simulink model "DetailedModel"  (R2024b)
settings: Solver=ode23t  StartTime=0.0  StopTime=0.2  MaxStep=1e-6  RelTol=1e-4
InitFcn:
  | ModelParameters
undefined symbols (not defined in the file or in its folder): ABR, abr, dc, dc_vs, h_BTU, inv, L, setpoint, Setpoint_Harmonic_L1, time, ts, Ts_RMS
libraries: spsThreePhaseSeriesRLCBranchLib x17, spsGroundLib x14, spsControlledVoltageSourceLib x11, spsThreePhaseVIMeasurementLib x8, spsSeriesRLCBranchLib x7, eePwmGenerator x6, spsCurrentMeasurementLib x4, spsVoltageMeasurementLib x4, spsControlledCurrentSourceLib x3, eePowerMeasurement x3, spsUniversalBridgeLib x2, spsThreePhaseBreakerLib x1
(part 2 of 3)

== system DetailedModel/ powerline/ 10 km ==
  note: L1
  note: L2
  Ground : spsGroundLib/Ground  LConnTagsString=a
  Three-Phase Series RLC Branch1 : spsThreePhaseSeriesRLCBranchLib/Three-Phase Series RLC Branch  LConnTagsString=A|B|C  RConnTagsString=A|B|C  BranchType=RL  Resistance=R  Inductance=L  Capacitance=1e-6  Measurements=None
  Three-Phase Series RLC Branch2 : spsThreePhaseSeriesRLCBranchLib/Three-Phase Series RLC Branch  LConnTagsString=A|B|C  RConnTagsString=A|B|C  BranchType=C  Resistance=inv.RC  Inductance=13e-6  Capacitance=C  Measurements=None
  Three-Phase Series RLC Branch3 : spsThreePhaseSeriesRLCBranchLib/Three-Phase Series RLC Branch  LConnTagsString=A|B|C  RConnTagsString=A|B|C  BranchType=C  Resistance=inv.RC  Inductance=13e-6  Capacitance=C  Measurements=None
  A1 : PMIOPort  Side=Left
  B1 : PMIOPort  Port=2  Side=Left
  C1 : PMIOPort  Port=3  Side=Left
  A2 : PMIOPort  Port=4  Side=Right
  B2 : PMIOPort  Port=5  Side=Right
  C2 : PMIOPort  Port=6  Side=Right
  connections:
  Three-Phase Series RLC Branch3/RConn1 -- Three-Phase Series RLC Branch3/RConn2 -- Three-Phase Series RLC Branch3/RConn3 -- Ground/LConn1 -- Three-Phase Series RLC Branch2/RConn1 -- Three-Phase Series RLC Branch2/RConn3 -- Three-Phase Series RLC Branch2/RConn2
  Three-Phase Series RLC Branch3/LConn1 -- Three-Phase Series RLC Branch1/LConn3 -- C1/RConn1
  C2/RConn1 -- Three-Phase Series RLC Branch2/LConn1 -- Three-Phase Series RLC Branch1/RConn3
  Three-Phase Series RLC Branch3/LConn2 -- Three-Phase Series RLC Branch1/LConn2 -- B1/RConn1
  B2/RConn1 -- Three-Phase Series RLC Branch1/RConn2 -- Three-Phase Series RLC Branch2/LConn2
  Three-Phase Series RLC Branch3/LConn3 -- Three-Phase Series RLC Branch1/LConn1 -- A1/RConn1
  A2/RConn1 -- Three-Phase Series RLC Branch1/RConn1 -- Three-Phase Series RLC Branch2/LConn3

== system DetailedModel/ powerline/ 15 km ==
  note: L2
  note: L1
  Ground : spsGroundLib/Ground  LConnTagsString=a
  Three-Phase Series RLC Branch1 : spsThreePhaseSeriesRLCBranchLib/Three-Phase Series RLC Branch  LConnTagsString=A|B|C  RConnTagsString=A|B|C  BranchType=RL  Resistance=R  Inductance=L  Capacitance=1e-6  Measurements=None
  Three-Phase Series RLC Branch2 : spsThreePhaseSeriesRLCBranchLib/Three-Phase Series RLC Branch  LConnTagsString=A|B|C  RConnTagsString=A|B|C  BranchType=C  Resistance=inv.RC  Inductance=13e-6  Capacitance=C  Measurements=None
  Three-Phase Series RLC Branch3 : spsThreePhaseSeriesRLCBranchLib/Three-Phase Series RLC Branch  LConnTagsString=A|B|C  RConnTagsString=A|B|C  BranchType=C  Resistance=inv.RC  Inductance=13e-6  Capacitance=C  Measurements=None
  A1 : PMIOPort  Side=Left
  B1 : PMIOPort  Port=2  Side=Left
  C1 : PMIOPort  Port=3  Side=Left
  A2 : PMIOPort  Port=4  Side=Right
  B2 : PMIOPort  Port=5  Side=Right
  C2 : PMIOPort  Port=6  Side=Right
  connections:
  Three-Phase Series RLC Branch2/LConn3 -- Three-Phase Series RLC Branch1/RConn1 -- A2/RConn1
  A1/RConn1 -- Three-Phase Series RLC Branch1/LConn1 -- Three-Phase Series RLC Branch3/LConn3
  Three-Phase Series RLC Branch2/LConn2 -- Three-Phase Series RLC Branch1/RConn2 -- B2/RConn1
  B1/RConn1 -- Three-Phase Series RLC Branch1/LConn2 -- Three-Phase Series RLC Branch3/LConn2
  Three-Phase Series RLC Branch1/RConn3 -- Three-Phase Series RLC Branch2/LConn1 -- C2/RConn1
  C1/RConn1 -- Three-Phase Series RLC Branch1/LConn3 -- Three-Phase Series RLC Branch3/LConn1
  Three-Phase Series RLC Branch2/RConn2 -- Three-Phase Series RLC Branch2/RConn3 -- Three-Phase Series RLC Branch2/RConn1 -- Ground/LConn1 -- Three-Phase Series RLC Branch3/RConn3 -- Three-Phase Series RLC Branch3/RConn2 -- Three-Phase Series RLC Branch3/RConn1

== system DetailedModel/ABR_Control/deactive ==
  V_dc : Inport
  V_grid_in : Inport  Port=2
  I_abr_in : Inport  Port=3
  DC_PosNeg : Inport  Port=4
  Enable_Control : Inport  Port=5
  Constant : Constant  Value=[0,0,0]
  Terminator{,1..4} (5 alike) : Terminator
  V_abr_ref : Outport
  wires:
  V_dc/1 -> Terminator/1
  V_grid_in/1 -> Terminator1/1
  Enable_Control/1 -> Terminator4/1
  DC_PosNeg/1 -> Terminator3/1
  I_abr_in/1 -> Terminator2/1
  Constant/1 -> V_abr_ref/1

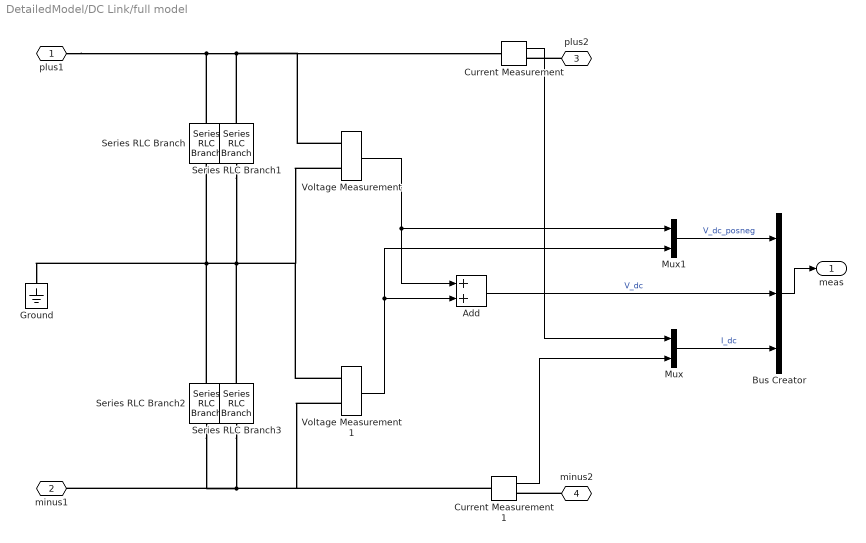
== system DetailedModel/DC Link/full model ==
  Add : Sum
  Bus Creator : BusCreator  Inputs=3
  Current Measurement : spsCurrentMeasurementLib/Current Measurement  PhasorSimulation=off  OutputType=Complex  PSBequivalent=0
  Current Measurement1 : spsCurrentMeasurementLib/Current Measurement  PhasorSimulation=off  OutputType=Complex  PSBequivalent=0
  Ground : spsGroundLib/Ground  LConnTagsString=a
  Mux : Mux  Inputs=2
  Mux1 : Mux  Inputs=2
  Series RLC Branch : spsSeriesRLCBranchLib/Series RLC Branch  LConnTagsString=__new0  RConnTagsString=__new0  BranchType=C  Resistance=1  Inductance=1e-3  SetiL0=off  InitialCurrent=0  Capacitance=dc.C  Setx0=on  InitialVoltage=ABR.Setpoint.Vdc_Enable/2  Measurements=None
  Series RLC Branch1 : spsSeriesRLCBranchLib/Series RLC Branch  LConnTagsString=__new0  RConnTagsString=__new0  BranchType=R  Resistance=dc.R  Inductance=1e-3  SetiL0=off  InitialCurrent=0  Capacitance=4700e-6  Setx0=on  InitialVoltage=325  Measurements=None
  Series RLC Branch2 : spsSeriesRLCBranchLib/Series RLC Branch  LConnTagsString=__new0  RConnTagsString=__new0  BranchType=C  Resistance=1  Inductance=1e-3  SetiL0=off  InitialCurrent=0  Capacitance=dc.C  Setx0=on  InitialVoltage=ABR.Setpoint.Vdc_Enable/2  Measurements=None
  Series RLC Branch3 : spsSeriesRLCBranchLib/Series RLC Branch  LConnTagsString=__new0  RConnTagsString=__new0  BranchType=R  Resistance=dc.R  Inductance=1e-3  SetiL0=off  InitialCurrent=0  Capacitance=4700e-6  Setx0=on  InitialVoltage=325  Measurements=None
  Voltage Measurement : spsVoltageMeasurementLib/Voltage Measurement  PhasorSimulation=off  OutputType=Complex  PSBequivalent=0
  Voltage Measurement1 : spsVoltageMeasurementLib/Voltage Measurement  PhasorSimulation=off  OutputType=Complex  PSBequivalent=0
  plus1 : PMIOPort  Side=Left
  minus1 : PMIOPort  Port=2  Side=Left
  plus2 : PMIOPort  Port=3  Side=Right
  minus2 : PMIOPort  Port=4  Side=Right
  meas : Outport
  wires:
  Add/1 -> Bus Creator/2  "V_dc"
  Bus Creator/1 -> meas/1
  Mux1/1 -> Bus Creator/1  "V_dc_posneg"
  Voltage Measurement1/1 -> Mux1/2, Add/2
  Voltage Measurement/1 -> Mux1/1, Add/1
  Current Measurement/1 -> Mux/1
  Current Measurement1/1 -> Mux/2
  Mux/1 -> Bus Creator/3  "I_dc"
  connections:
  plus1/RConn1 -- Series RLC Branch/LConn1 -- Voltage Measurement/LConn1 -- Current Measurement/LConn1 -- Series RLC Branch1/LConn1
  Current Measurement1/LConn1 -- Voltage Measurement1/LConn2 -- Series RLC Branch2/RConn1 -- minus1/RConn1 -- Series RLC Branch3/RConn1
  Series RLC Branch2/LConn1 -- Series RLC Branch/RConn1 -- Ground/LConn1 -- Voltage Measurement/LConn2 -- Voltage Measurement1/LConn1 -- Series RLC Branch3/LConn1 -- Series RLC Branch1/RConn1
  plus2/RConn1 -- Current Measurement/RConn1
  minus2/RConn1 -- Current Measurement1/RConn1

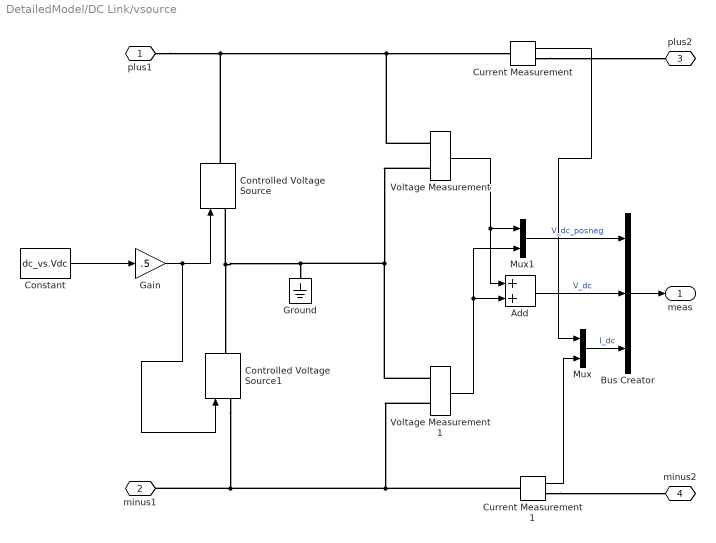
== system DetailedModel/DC Link/vsource ==
  Add : Sum
  Bus Creator : BusCreator  Inputs=3
  Constant : Constant  Value=dc_vs.Vdc
  Controlled Voltage Source : spsControlledVoltageSourceLib/Controlled Voltage Source  Initialize=on  Source_Type=AC  Amplitude=0  Phase=0  Frequency=0  Measurements=None
  Controlled Voltage Source1 : spsControlledVoltageSourceLib/Controlled Voltage Source  Initialize=on  Source_Type=AC  Amplitude=0  Phase=0  Frequency=0  Measurements=None
  Current Measurement : spsCurrentMeasurementLib/Current Measurement  PhasorSimulation=off  OutputType=Complex  PSBequivalent=0
  Current Measurement1 : spsCurrentMeasurementLib/Current Measurement  PhasorSimulation=off  OutputType=Complex  PSBequivalent=0
  Gain : Gain  Gain=.5
  Ground : spsGroundLib/Ground  LConnTagsString=a
  Mux : Mux  Inputs=2
  Mux1 : Mux  Inputs=2
  Voltage Measurement : spsVoltageMeasurementLib/Voltage Measurement  PhasorSimulation=off  OutputType=Complex  PSBequivalent=0
  Voltage Measurement1 : spsVoltageMeasurementLib/Voltage Measurement  PhasorSimulation=off  OutputType=Complex  PSBequivalent=0
  plus1 : PMIOPort  Side=Left
  minus1 : PMIOPort  Port=2  Side=Left
  plus2 : PMIOPort  Port=3  Side=Right
  minus2 : PMIOPort  Port=4  Side=Right
  meas : Outport
  wires:
  Add/1 -> Bus Creator/2  "V_dc"
  Voltage Measurement1/1 -> Mux1/2, Add/2
  Voltage Measurement/1 -> Mux1/1, Add/1
  Bus Creator/1 -> meas/1
  Mux1/1 -> Bus Creator/1  "V_dc_posneg"
  Gain/1 -> Controlled Voltage Source/1, Controlled Voltage Source1/1
  Constant/1 -> Gain/1
  Mux/1 -> Bus Creator/3  "I_dc"
  Current Measurement/1 -> Mux/1
  Current Measurement1/1 -> Mux/2
  connections:
  plus1/RConn1 -- Controlled Voltage Source/RConn1 -- Current Measurement/LConn1 -- Voltage Measurement/LConn1
  Current Measurement1/LConn1 -- Voltage Measurement1/LConn2 -- Controlled Voltage Source1/LConn1 -- minus1/RConn1
  Controlled Voltage Source/LConn1 -- Voltage Measurement/LConn2 -- Voltage Measurement1/LConn1 -- Ground/LConn1 -- Controlled Voltage Source1/RConn1
  Current Measurement/RConn1 -- plus2/RConn1
  Current Measurement1/RConn1 -- minus2/RConn1

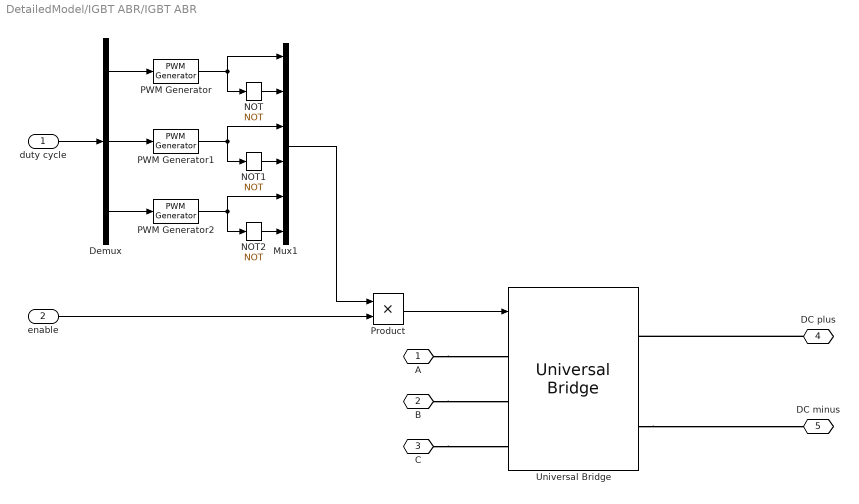
== system DetailedModel/IGBT ABR/IGBT ABR ==
  duty cycle : Inport
  enable : Inport  Port=2
  Demux : Demux  Outputs=3
  Mux1 : Mux  Inputs=6
  NOT : Logic  Operator=NOT  IconShape=distinctive  AllPortsSameDT=off  OutDataTypeStr=boolean
  NOT1 : Logic  Operator=NOT  IconShape=distinctive  AllPortsSameDT=off  OutDataTypeStr=boolean
  NOT2 : Logic  Operator=NOT  IconShape=distinctive  AllPortsSameDT=off  OutDataTypeStr=boolean
  PWM Generator : eePwmGenerator/PWM Generator  CarrCount=Up  Tper=abr.h_PWM  Tdelay=0  Ts=0
  PWM Generator1 : eePwmGenerator/PWM Generator  CarrCount=Up  Tper=abr.h_PWM  Tdelay=0  Ts=0
  PWM Generator2 : eePwmGenerator/PWM Generator  CarrCount=Up  Tper=abr.h_PWM  Tdelay=0  Ts=0
  Product : Product
  Universal Bridge : spsUniversalBridgeLib/Universal Bridge  Arms=3  SnubberResistance=1e5  SnubberCapacitance=inf  Device=IGBT / Diodes  Ron=1e-3  Lon=0  ForwardVoltages="[  0  0  ]"  ForwardVoltage=0  GTOparameters=[ 10e-6 , 20e-6 ]  IGBTparameters=[ 1e-6 , 2e-6 ]  Measurements=None  Measurements_2=None  converterType=Rectifier
  A : PMIOPort  Side=Left
  B : PMIOPort  Port=2  Side=Left
  C : PMIOPort  Port=3  Side=Left
  DC plus : PMIOPort  Port=4  Side=Right
  DC minus : PMIOPort  Port=5  Side=Right
  wires:
  enable/1 -> Product/2
  Demux/1 -> PWM Generator/1
  Mux1/1 -> Product/1
  Demux/3 -> PWM Generator2/1
  NOT2/1 -> Mux1/6
  PWM Generator2/1 -> NOT2/1, Mux1/5
  Demux/2 -> PWM Generator1/1
  PWM Generator1/1 -> NOT1/1, Mux1/3
  NOT1/1 -> Mux1/4
  NOT/1 -> Mux1/2
  PWM Generator/1 -> NOT/1, Mux1/1
  duty cycle/1 -> Demux/1
  Product/1 -> Universal Bridge/1
  connections:
  Universal Bridge/RConn2 -- DC minus/RConn1
  C/RConn1 -- Universal Bridge/LConn3
  A/RConn1 -- Universal Bridge/LConn1
  B/RConn1 -- Universal Bridge/LConn2
  DC plus/RConn1 -- Universal Bridge/RConn1

== system DetailedModel/IGBT ABR/deactivate ==
  duty cycle : Inport
  enable : Inport  Port=2
  Terminator : Terminator
  Terminator1 : Terminator
  A : PMIOPort  Side=Left
  B : PMIOPort  Port=2  Side=Left
  C : PMIOPort  Port=3  Side=Left
  DC plus : PMIOPort  Port=4  Side=Right
  DC minus : PMIOPort  Port=5  Side=Right
  wires:
  duty cycle/1 -> Terminator/1
  enable/1 -> Terminator1/1

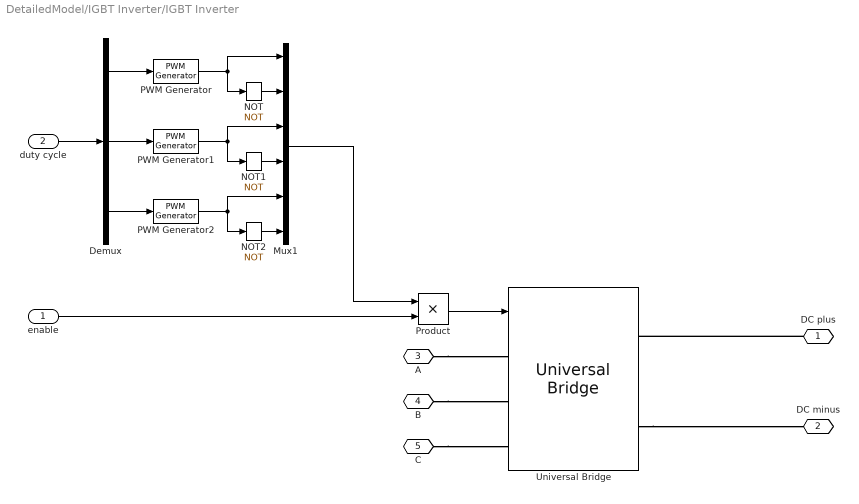
== system DetailedModel/IGBT Inverter/IGBT Inverter ==
  enable : Inport
  duty cycle : Inport  Port=2
  Demux : Demux  Outputs=3
  Mux1 : Mux  Inputs=6
  NOT : Logic  Operator=NOT  IconShape=distinctive  AllPortsSameDT=off  OutDataTypeStr=boolean
  NOT1 : Logic  Operator=NOT  IconShape=distinctive  AllPortsSameDT=off  OutDataTypeStr=boolean
  NOT2 : Logic  Operator=NOT  IconShape=distinctive  AllPortsSameDT=off  OutDataTypeStr=boolean
  PWM Generator : eePwmGenerator/PWM Generator  CarrCount=Up  Tper=inv.h_PWM  Tdelay=0  Ts=0
  PWM Generator1 : eePwmGenerator/PWM Generator  CarrCount=Up  Tper=inv.h_PWM  Tdelay=0  Ts=0
  PWM Generator2 : eePwmGenerator/PWM Generator  CarrCount=Up  Tper=inv.h_PWM  Tdelay=0  Ts=0
  Product : Product
  Universal Bridge : spsUniversalBridgeLib/Universal Bridge  Arms=3  SnubberResistance=1e5  SnubberCapacitance=inf  Device=IGBT / Diodes  Ron=1e-3  Lon=0  ForwardVoltages="[  0  0  ]"  ForwardVoltage=0  GTOparameters=[ 10e-6 , 20e-6 ]  IGBTparameters=[ 1e-6 , 2e-6 ]  Measurements=None  Measurements_2=None  converterType=Rectifier
  DC plus : PMIOPort  Side=Left
  DC minus : PMIOPort  Port=2  Side=Left
  A : PMIOPort  Port=3  Side=Right
  B : PMIOPort  Port=4  Side=Right
  C : PMIOPort  Port=5  Side=Right
  wires:
  duty cycle/1 -> Demux/1
  PWM Generator/1 -> Mux1/1, NOT/1
  NOT/1 -> Mux1/2
  NOT1/1 -> Mux1/4
  PWM Generator1/1 -> Mux1/3, NOT1/1
  Demux/2 -> PWM Generator1/1
  PWM Generator2/1 -> Mux1/5, NOT2/1
  NOT2/1 -> Mux1/6
  Demux/3 -> PWM Generator2/1
  Mux1/1 -> Product/1
  Demux/1 -> PWM Generator/1
  Product/1 -> Universal Bridge/1
  enable/1 -> Product/2
  connections:
  DC plus/RConn1 -- Universal Bridge/RConn1
  B/RConn1 -- Universal Bridge/LConn2
  A/RConn1 -- Universal Bridge/LConn1
  C/RConn1 -- Universal Bridge/LConn3
  Universal Bridge/RConn2 -- DC minus/RConn1

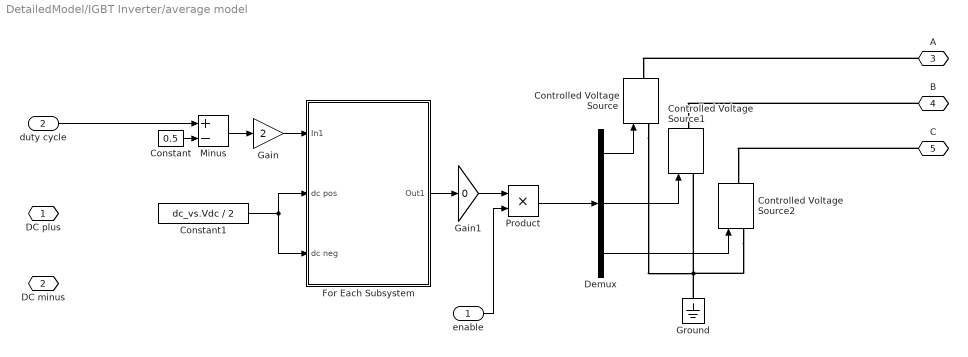
== system DetailedModel/IGBT Inverter/average model ==
  enable : Inport
  duty cycle : Inport  Port=2
  Constant : Constant  Value=0.5
  Constant1 : Constant  Value=dc_vs.Vdc / 2
  Controlled Voltage Source : spsControlledVoltageSourceLib/Controlled Voltage Source  Initialize=on  Source_Type=AC  Amplitude=0  Phase=0  Frequency=0  Measurements=None
  Controlled Voltage Source1 : spsControlledVoltageSourceLib/Controlled Voltage Source  Initialize=on  Source_Type=AC  Amplitude=0  Phase=0  Frequency=0  Measurements=None
  Controlled Voltage Source2 : spsControlledVoltageSourceLib/Controlled Voltage Source  Initialize=on  Source_Type=AC  Amplitude=0  Phase=0  Frequency=0  Measurements=None
  Demux : Demux  Outputs=3
  For Each Subsystem : Subsystem  TreatAsAtomicUnit=on
  Gain : Gain  Gain=2
  Gain1 : Gain  Gain=0
  Ground : spsGroundLib/Ground  LConnTagsString=a
  Minus : Sum  Inputs=+-
  Product : Product
  DC plus : PMIOPort  Side=Left
  DC minus : PMIOPort  Port=2  Side=Left
  A : PMIOPort  Port=3  Side=Right
  B : PMIOPort  Port=4  Side=Right
  C : PMIOPort  Port=5  Side=Right
  wires:
  enable/1 -> Product/2
  duty cycle/1 -> Minus/1
  Constant/1 -> Minus/2
  Minus/1 -> Gain/1
  Gain/1 -> For Each Subsystem/1(In1)
  Constant1/1 -> For Each Subsystem/2(dc pos), For Each Subsystem/3(dc neg)
  Demux/2 -> Controlled Voltage Source1/1
  Demux/3 -> Controlled Voltage Source2/1
  For Each Subsystem/1(Out1) -> Gain1/1
  Product/1 -> Demux/1
  Demux/1 -> Controlled Voltage Source/1
  Gain1/1 -> Product/1
  connections:
  Controlled Voltage Source/LConn1 -- Ground/LConn1 -- Controlled Voltage Source1/LConn1 -- Controlled Voltage Source2/LConn1
  B/RConn1 -- Controlled Voltage Source1/RConn1
  C/RConn1 -- Controlled Voltage Source2/RConn1
  A/RConn1 -- Controlled Voltage Source/RConn1

== system DetailedModel/Voltage Source/Voltage Source ==
  3ph in : Inport
  Controlled Voltage Source : spsControlledVoltageSourceLib/Controlled Voltage Source  Initialize=on  Source_Type=AC  Amplitude=0  Phase=0  Frequency=0  Measurements=None
  Controlled Voltage Source1 : spsControlledVoltageSourceLib/Controlled Voltage Source  Initialize=on  Source_Type=AC  Amplitude=0  Phase=0  Frequency=0  Measurements=None
  Controlled Voltage Source2 : spsControlledVoltageSourceLib/Controlled Voltage Source  Initialize=on  Source_Type=AC  Amplitude=0  Phase=0  Frequency=0  Measurements=None
  Demux : Demux  Outputs=3
  Ground : spsGroundLib/Ground  LConnTagsString=a
  a : PMIOPort  Side=Right
  b : PMIOPort  Port=2  Side=Right
  c : PMIOPort  Port=3  Side=Right
  wires:
  3ph in/1 -> Demux/1
  Demux/3 -> Controlled Voltage Source2/1
  Demux/2 -> Controlled Voltage Source1/1
  Demux/1 -> Controlled Voltage Source/1
  connections:
  Controlled Voltage Source2/RConn1 -- c/RConn1
  b/RConn1 -- Controlled Voltage Source1/RConn1
  Controlled Voltage Source/RConn1 -- a/RConn1
  Ground/LConn1 -- Controlled Voltage Source1/LConn1 -- Controlled Voltage Source2/LConn1 -- Controlled Voltage Source/LConn1

== system DetailedModel/Voltage Source/deactive ==
  3ph in : Inport
  Ground : spsGroundLib/Ground  LConnTagsString=a
  Terminator : Terminator
  a : PMIOPort  Side=Right
  b : PMIOPort  Port=2  Side=Right
  c : PMIOPort  Port=3  Side=Right
  wires:
  3ph in/1 -> Terminator/1
  connections:
  c/RConn1 -- b/RConn1 -- a/RConn1 -- Ground/LConn1

== system DetailedModel/input LCL/deactive ==
  Bus Creator : BusCreator  Inputs=6
  Constant{,1..5} (6 alike) : Constant  Value=[0,0,0]
  A1 : PMIOPort  Side=Left
  B1 : PMIOPort  Port=2  Side=Left
  C1 : PMIOPort  Port=3  Side=Left
  A2 : PMIOPort  Port=4  Side=Right
  B2 : PMIOPort  Port=5  Side=Right
  C2 : PMIOPort  Port=6  Side=Right
  meas : Outport
  wires:
  Bus Creator/1 -> meas/1
  Constant5/1 -> Bus Creator/6  "abr_I_C"
  Constant4/1 -> Bus Creator/5  "abr_U_C"
  Constant3/1 -> Bus Creator/4  "abr_I_L2"
  Constant2/1 -> Bus Creator/3  "abr_U_out"
  Constant1/1 -> Bus Creator/2  "abr_I_L1"
  Constant/1 -> Bus Creator/1  "abr_U_in"
  connections:
  A1/RConn1 -- A2/RConn1
  C2/RConn1 -- C1/RConn1
  B1/RConn1 -- B2/RConn1

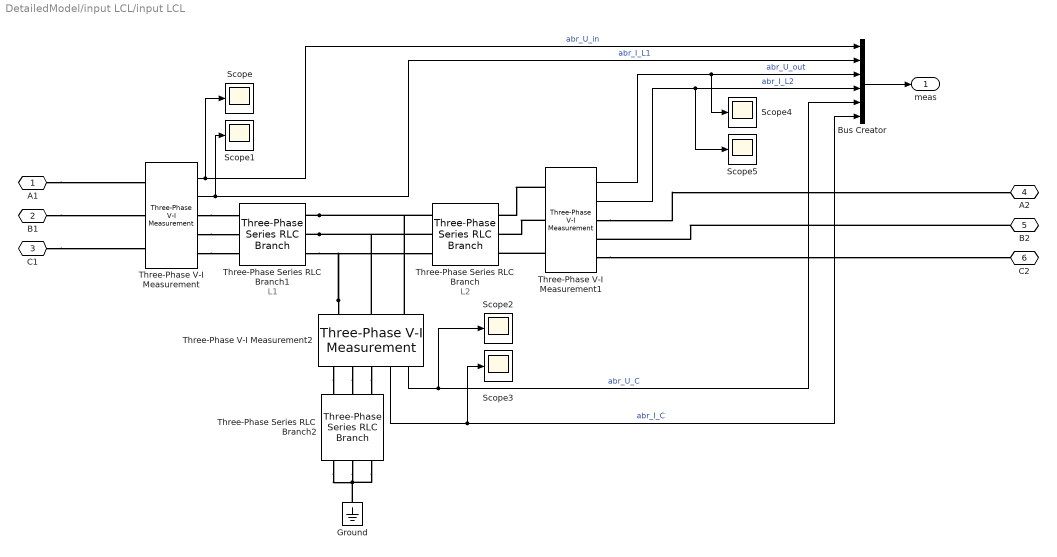
== system DetailedModel/input LCL/input LCL ==
  note: L1
  note: L2
  Bus Creator : BusCreator  Inputs=6
  Ground : spsGroundLib/Ground  LConnTagsString=a
  Scope{,1..5} (6 alike) : Scope
  Three-Phase Series RLC Branch : spsThreePhaseSeriesRLCBranchLib/Three-Phase Series RLC Branch  LConnTagsString=A|B|C  RConnTagsString=A|B|C  BranchType=RL  Resistance=abr.R2  Inductance=abr.L2  Capacitance=1e-6  Measurements=None
  Three-Phase Series RLC Branch1 : spsThreePhaseSeriesRLCBranchLib/Three-Phase Series RLC Branch  LConnTagsString=A|B|C  RConnTagsString=A|B|C  BranchType=RL  Resistance=abr.R1  Inductance=abr.L1  Capacitance=1e-6  Measurements=None
  Three-Phase Series RLC Branch2 : spsThreePhaseSeriesRLCBranchLib/Three-Phase Series RLC Branch  LConnTagsString=A|B|C  RConnTagsString=A|B|C  BranchType=RC  Resistance=abr.RC  Inductance=13e-6  Capacitance=abr.C  Measurements=None
  Three-Phase V-I Measurement : spsThreePhaseVIMeasurementLib/Three-Phase V-I Measurement  VoltageMeasurement=phase-to-ground  SetLabelV=off  LabelV=Vabc  Vpu=off  VpuLL=off  CurrentMeasurement=yes  SetLabelI=off  LabelI=Iabc  Ipu=off  Pbase=100e6  Vbase=500e3  OutputType=Complex  PhasorSimulation=off  PSBequivalent=0
  Three-Phase V-I Measurement1 : spsThreePhaseVIMeasurementLib/Three-Phase V-I Measurement  VoltageMeasurement=phase-to-ground  SetLabelV=off  LabelV=Vabc  Vpu=off  VpuLL=off  CurrentMeasurement=yes  SetLabelI=off  LabelI=Iabc  Ipu=off  Pbase=100e6  Vbase=500e3  OutputType=Complex  PhasorSimulation=off  PSBequivalent=0
  Three-Phase V-I Measurement2 : spsThreePhaseVIMeasurementLib/Three-Phase V-I Measurement  VoltageMeasurement=phase-to-ground  SetLabelV=off  LabelV=Vabc  Vpu=off  VpuLL=off  CurrentMeasurement=yes  SetLabelI=off  LabelI=Iabc  Ipu=off  Pbase=100e6  Vbase=500e3  OutputType=Complex  PhasorSimulation=off  PSBequivalent=0
  A1 : PMIOPort  Side=Left
  B1 : PMIOPort  Port=2  Side=Left
  C1 : PMIOPort  Port=3  Side=Left
  A2 : PMIOPort  Port=4  Side=Right
  B2 : PMIOPort  Port=5  Side=Right
  C2 : PMIOPort  Port=6  Side=Right
  meas : Outport
  wires:
  Bus Creator/1 -> meas/1
  Three-Phase V-I Measurement2/2 -> Scope3/1, Bus Creator/6  "abr_I_C"
  Three-Phase V-I Measurement2/1 -> Scope2/1, Bus Creator/5  "abr_U_C"
  Three-Phase V-I Measurement1/2 -> Scope5/1, Bus Creator/4  "abr_I_L2"
  Three-Phase V-I Measurement1/1 -> Scope4/1, Bus Creator/3  "abr_U_out"
  Three-Phase V-I Measurement/2 -> Scope1/1, Bus Creator/2  "abr_I_L1"
  Three-Phase V-I Measurement/1 -> Scope/1, Bus Creator/1  "abr_U_in"
  connections:
  Three-Phase Series RLC Branch2/RConn3 -- Ground/LConn1 -- Three-Phase Series RLC Branch2/RConn2 -- Three-Phase Series RLC Branch2/RConn1
  Three-Phase V-I Measurement2/RConn3 -- Three-Phase Series RLC Branch2/LConn1
  Three-Phase V-I Measurement1/LConn1 -- Three-Phase Series RLC Branch/RConn1
  Three-Phase V-I Measurement/RConn3 -- Three-Phase Series RLC Branch1/LConn3
  Three-Phase V-I Measurement1/RConn1 -- A2/RConn1
  Three-Phase V-I Measurement2/LConn3 -- Three-Phase Series RLC Branch/LConn3 -- Three-Phase Series RLC Branch1/RConn3
  C1/RConn1 -- Three-Phase V-I Measurement/LConn3
  Three-Phase V-I Measurement1/LConn3 -- Three-Phase Series RLC Branch/RConn3
  Three-Phase V-I Measurement/RConn2 -- Three-Phase Series RLC Branch1/LConn2
  Three-Phase Series RLC Branch1/RConn2 -- Three-Phase Series RLC Branch/LConn2 -- Three-Phase V-I Measurement2/LConn2
  A1/RConn1 -- Three-Phase V-I Measurement/LConn1
  Three-Phase V-I Measurement2/RConn1 -- Three-Phase Series RLC Branch2/LConn3
  Three-Phase V-I Measurement/RConn1 -- Three-Phase Series RLC Branch1/LConn1
  Three-Phase V-I Measurement1/LConn2 -- Three-Phase Series RLC Branch/RConn2
  Three-Phase Series RLC Branch1/RConn1 -- Three-Phase Series RLC Branch/LConn1 -- Three-Phase V-I Measurement2/LConn1
  Three-Phase V-I Measurement2/RConn2 -- Three-Phase Series RLC Branch2/LConn2
  B1/RConn1 -- Three-Phase V-I Measurement/LConn2
  B2/RConn1 -- Three-Phase V-I Measurement1/RConn2
  Three-Phase V-I Measurement1/RConn3 -- C2/RConn1

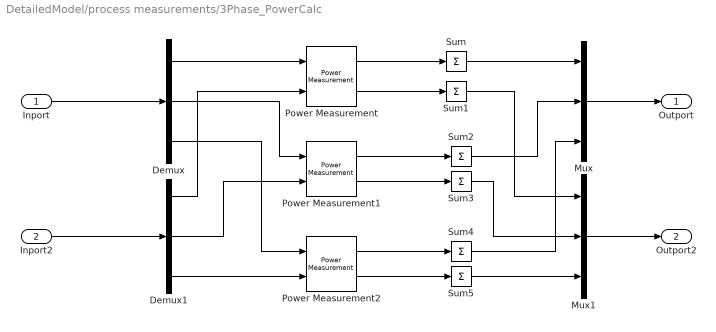
== system DetailedModel/process measurements/3Phase_PowerCalc ==
  Inport : Inport
  Inport2 : Inport  Port=2
  Demux : Demux  Outputs=3
  Demux1 : Demux  Outputs=3
  Mux : Mux  Inputs=3
  Mux1 : Mux  Inputs=3
  Power Measurement : eePowerMeasurement/Power Measurement  LabelModeActiveChoice=Discrete  F=50  K=[0 1 2 3]  Ts=Ts_RMS
  Power Measurement1 : eePowerMeasurement/Power Measurement  LabelModeActiveChoice=Discrete  F=50  K=[0 1 2 3]  Ts=Ts_RMS
  Power Measurement2 : eePowerMeasurement/Power Measurement  LabelModeActiveChoice=Discrete  F=50  K=[0 1 2 3]  Ts=Ts_RMS
  Sum{,1..5} (6 alike) : Sum  Inputs=+
  Outport : Outport
  Outport2 : Outport  Port=2
  wires:
  Demux/1 -> Power Measurement/1
  Demux/2 -> Power Measurement1/1
  Inport/1 -> Demux/1
  Power Measurement/2 -> Sum1/1
  Inport2/1 -> Demux1/1
  Power Measurement/1 -> Sum/1
  Demux/3 -> Power Measurement2/1
  Demux1/1 -> Power Measurement/2
  Demux1/2 -> Power Measurement1/2
  Demux1/3 -> Power Measurement2/2
  Power Measurement1/1 -> Sum2/1
  Power Measurement1/2 -> Sum3/1
  Power Measurement2/2 -> Sum5/1
  Power Measurement2/1 -> Sum4/1
  Sum/1 -> Mux/1
  Sum2/1 -> Mux/2
  Sum4/1 -> Mux/3
  Sum1/1 -> Mux1/1
  Sum3/1 -> Mux1/2
  Sum5/1 -> Mux1/3
  Mux1/1 -> Outport2/1
  Mux/1 -> Outport/1

== system DetailedModel/process measurements/DMA Averaging ==
  In1 : Inport
  Demux : Demux  Outputs=3
  Mux : Mux  Inputs=3
  Subsystem Reference1 : Subsystem  ReferencedSubsystem=DMA_frame_average  samplerate=h_BTU  framesize=DMA_framesize
  Subsystem Reference2 : Subsystem  ReferencedSubsystem=DMA_frame_average  samplerate=h_BTU  framesize=DMA_framesize
  Subsystem Reference3 : Subsystem  ReferencedSubsystem=DMA_frame_average  samplerate=h_BTU  framesize=DMA_framesize
  Out1 : Outport
  wires:
  Mux/1 -> Out1/1
  Demux/3 -> Subsystem Reference3/1
  Demux/2 -> Subsystem Reference2/1
  Subsystem Reference2/1 -> Mux/2
  In1/1 -> Demux/1
  Subsystem Reference1/1 -> Mux/1
  Subsystem Reference3/1 -> Mux/3
  Demux/1 -> Subsystem Reference1/1

== system DetailedModel/process measurements/DMA Averaging1 ==
  In1 : Inport
  Demux : Demux  Outputs=3
  Mux : Mux  Inputs=3
  Subsystem Reference1 : Subsystem  ReferencedSubsystem=DMA_frame_average  samplerate=h_BTU  framesize=DMA_framesize
  Subsystem Reference2 : Subsystem  ReferencedSubsystem=DMA_frame_average  samplerate=h_BTU  framesize=DMA_framesize
  Subsystem Reference3 : Subsystem  ReferencedSubsystem=DMA_frame_average  samplerate=h_BTU  framesize=DMA_framesize
  u : Outport
  wires:
  Demux/1 -> Subsystem Reference1/1
  Subsystem Reference3/1 -> Mux/3
  Subsystem Reference1/1 -> Mux/1
  In1/1 -> Demux/1
  Subsystem Reference2/1 -> Mux/2
  Demux/2 -> Subsystem Reference2/1
  Demux/3 -> Subsystem Reference3/1
  Mux/1 -> u/1

== system DetailedModel/process measurements/DMA Averaging11 ==
  In1 : Inport
  Demux : Demux  Outputs=3
  Mux : Mux  Inputs=3
  Subsystem Reference1 : Subsystem  ReferencedSubsystem=DMA_frame_average  samplerate=h_BTU  framesize=DMA_framesize
  Subsystem Reference2 : Subsystem  ReferencedSubsystem=DMA_frame_average  samplerate=h_BTU  framesize=DMA_framesize
  Subsystem Reference3 : Subsystem  ReferencedSubsystem=DMA_frame_average  samplerate=h_BTU  framesize=DMA_framesize
  Out1 : Outport
  wires:
  Demux/1 -> Subsystem Reference1/1
  Subsystem Reference3/1 -> Mux/3
  Subsystem Reference1/1 -> Mux/1
  In1/1 -> Demux/1
  Subsystem Reference2/1 -> Mux/2
  Demux/2 -> Subsystem Reference2/1
  Demux/3 -> Subsystem Reference3/1
  Mux/1 -> Out1/1

== system DetailedModel/process measurements/DMA Averaging12 ==
  In1 : Inport
  Demux : Demux  Outputs=3
  Mux : Mux  Inputs=3
  Scope : Scope  Commented=on  NumInputPorts=3
  Scope1 : Scope  Commented=on  NumInputPorts=3
  Scope2 : Scope  Commented=on  NumInputPorts=3
  Subsystem Reference1 : Subsystem  ReferencedSubsystem=DMA_frame_average  samplerate=h_BTU  framesize=DMA_framesize
  Subsystem Reference2 : Subsystem  ReferencedSubsystem=DMA_frame_average  samplerate=h_BTU  framesize=DMA_framesize
  Subsystem Reference3 : Subsystem  ReferencedSubsystem=DMA_frame_average  samplerate=h_BTU  framesize=DMA_framesize
  Zero-Order Hold : ZeroOrderHold  Commented=on  SampleTime=h_BTU
  Zero-Order Hold1 : ZeroOrderHold  Commented=on  SampleTime=h_BTU
  Zero-Order Hold2 : ZeroOrderHold  Commented=on  SampleTime=h_BTU
  Zero-Order Hold3 : ZeroOrderHold  Commented=on  SampleTime=h_BTU/10
  Zero-Order Hold4 : ZeroOrderHold  Commented=on  SampleTime=h_BTU/10
  Zero-Order Hold5 : ZeroOrderHold  Commented=on  SampleTime=h_BTU/10
  u : Outport
  wires:
  Mux/1 -> u/1
  In1/1 -> Demux/1
  Subsystem Reference1/1 -> Scope/3, Mux/1
  Zero-Order Hold/1 -> Scope/2
  Demux/1 -> Zero-Order Hold3/1, Zero-Order Hold/1, Subsystem Reference1/1
  Subsystem Reference2/1 -> Scope1/3, Mux/2
  Demux/2 -> Zero-Order Hold4/1, Zero-Order Hold1/1, Subsystem Reference2/1
  Zero-Order Hold1/1 -> Scope1/2
  Subsystem Reference3/1 -> Scope2/3, Mux/3
  Demux/3 -> Zero-Order Hold2/1, Zero-Order Hold5/1, Subsystem Reference3/1
  Zero-Order Hold2/1 -> Scope2/2
  Zero-Order Hold3/1 -> Scope/1
  Zero-Order Hold4/1 -> Scope1/1
  Zero-Order Hold5/1 -> Scope2/1

== system DetailedModel/process measurements/DMA Averaging13 ==
  In1 : Inport
  Demux : Demux  Outputs=3
  Mux : Mux  Inputs=3
  Subsystem Reference1 : Subsystem  ReferencedSubsystem=DMA_frame_average  samplerate=h_BTU  framesize=DMA_framesize
  Subsystem Reference2 : Subsystem  ReferencedSubsystem=DMA_frame_average  samplerate=h_BTU  framesize=DMA_framesize
  Subsystem Reference3 : Subsystem  ReferencedSubsystem=DMA_frame_average  samplerate=h_BTU  framesize=DMA_framesize
  u : Outport
  wires:
  Demux/1 -> Subsystem Reference1/1
  Subsystem Reference3/1 -> Mux/3
  Subsystem Reference1/1 -> Mux/1
  In1/1 -> Demux/1
  Subsystem Reference2/1 -> Mux/2
  Demux/2 -> Subsystem Reference2/1
  Demux/3 -> Subsystem Reference3/1
  Mux/1 -> u/1

== system DetailedModel/process measurements/DMA Averaging14 ==
  In1 : Inport
  Demux : Demux  Outputs=3
  Mux : Mux  Inputs=3
  Subsystem Reference1 : Subsystem  ReferencedSubsystem=DMA_frame_average  samplerate=h_BTU  framesize=DMA_framesize
  Subsystem Reference2 : Subsystem  ReferencedSubsystem=DMA_frame_average  samplerate=h_BTU  framesize=DMA_framesize
  Subsystem Reference3 : Subsystem  ReferencedSubsystem=DMA_frame_average  samplerate=h_BTU  framesize=DMA_framesize
  u : Outport
  wires:
  Mux/1 -> u/1
  Demux/3 -> Subsystem Reference3/1
  Demux/2 -> Subsystem Reference2/1
  Subsystem Reference2/1 -> Mux/2
  In1/1 -> Demux/1
  Subsystem Reference1/1 -> Mux/1
  Subsystem Reference3/1 -> Mux/3
  Demux/1 -> Subsystem Reference1/1

== system DetailedModel/process measurements/DMA Averaging15 ==
  In1 : Inport
  Demux : Demux  Outputs=3
  Mux : Mux  Inputs=3
  Subsystem Reference1 : Subsystem  ReferencedSubsystem=DMA_frame_average  samplerate=h_BTU  framesize=DMA_framesize
  Subsystem Reference2 : Subsystem  ReferencedSubsystem=DMA_frame_average  samplerate=h_BTU  framesize=DMA_framesize
  Subsystem Reference3 : Subsystem  ReferencedSubsystem=DMA_frame_average  samplerate=h_BTU  framesize=DMA_framesize
  u : Outport
  wires:
  Demux/1 -> Subsystem Reference1/1
  Subsystem Reference3/1 -> Mux/3
  Subsystem Reference1/1 -> Mux/1
  In1/1 -> Demux/1
  Subsystem Reference2/1 -> Mux/2
  Demux/2 -> Subsystem Reference2/1
  Demux/3 -> Subsystem Reference3/1
  Mux/1 -> u/1

== system DetailedModel/process measurements/DMA Averaging2 ==
  In1 : Inport
  Demux : Demux  Outputs=3
  Mux : Mux  Inputs=3
  Subsystem Reference1 : Subsystem  ReferencedSubsystem=DMA_frame_average  samplerate=h_BTU  framesize=DMA_framesize
  Subsystem Reference2 : Subsystem  ReferencedSubsystem=DMA_frame_average  samplerate=h_BTU  framesize=DMA_framesize
  Subsystem Reference3 : Subsystem  ReferencedSubsystem=DMA_frame_average  samplerate=h_BTU  framesize=DMA_framesize
  Out1 : Outport
  wires:
  Mux/1 -> Out1/1
  Demux/3 -> Subsystem Reference3/1
  Demux/2 -> Subsystem Reference2/1
  Subsystem Reference2/1 -> Mux/2
  In1/1 -> Demux/1
  Subsystem Reference1/1 -> Mux/1
  Subsystem Reference3/1 -> Mux/3
  Demux/1 -> Subsystem Reference1/1

== system DetailedModel/process measurements/DMA Averaging3 ==
  In1 : Inport
  Demux : Demux  Outputs=3
  Mux : Mux  Inputs=3
  Subsystem Reference1 : Subsystem  ReferencedSubsystem=DMA_frame_average  samplerate=h_BTU  framesize=DMA_framesize
  Subsystem Reference2 : Subsystem  ReferencedSubsystem=DMA_frame_average  samplerate=h_BTU  framesize=DMA_framesize
  Subsystem Reference3 : Subsystem  ReferencedSubsystem=DMA_frame_average  samplerate=h_BTU  framesize=DMA_framesize
  Out1 : Outport
  wires:
  Demux/1 -> Subsystem Reference1/1
  Subsystem Reference3/1 -> Mux/3
  Subsystem Reference1/1 -> Mux/1
  In1/1 -> Demux/1
  Subsystem Reference2/1 -> Mux/2
  Demux/2 -> Subsystem Reference2/1
  Demux/3 -> Subsystem Reference3/1
  Mux/1 -> Out1/1

== system DetailedModel/process measurements/DMA Averaging4 ==
  In1 : Inport
  Demux : Demux  Outputs=3
  Mux : Mux  Inputs=3
  Subsystem Reference1 : Subsystem  ReferencedSubsystem=DMA_frame_average  samplerate=h_BTU  framesize=DMA_framesize
  Subsystem Reference2 : Subsystem  ReferencedSubsystem=DMA_frame_average  samplerate=h_BTU  framesize=DMA_framesize
  Subsystem Reference3 : Subsystem  ReferencedSubsystem=DMA_frame_average  samplerate=h_BTU  framesize=DMA_framesize
  Out1 : Outport
  wires:
  Mux/1 -> Out1/1
  Demux/3 -> Subsystem Reference3/1
  Demux/2 -> Subsystem Reference2/1
  Subsystem Reference2/1 -> Mux/2
  In1/1 -> Demux/1
  Subsystem Reference1/1 -> Mux/1
  Subsystem Reference3/1 -> Mux/3
  Demux/1 -> Subsystem Reference1/1

== system DetailedModel/process measurements/DMA Averaging5 ==
  In1 : Inport
  Demux : Demux  Outputs=3
  Mux : Mux  Inputs=3
  Subsystem Reference1 : Subsystem  ReferencedSubsystem=DMA_frame_average  samplerate=h_BTU  framesize=DMA_framesize
  Subsystem Reference2 : Subsystem  ReferencedSubsystem=DMA_frame_average  samplerate=h_BTU  framesize=DMA_framesize
  Subsystem Reference3 : Subsystem  ReferencedSubsystem=DMA_frame_average  samplerate=h_BTU  framesize=DMA_framesize
  Out1 : Outport
  wires:
  Demux/1 -> Subsystem Reference1/1
  Subsystem Reference3/1 -> Mux/3
  Subsystem Reference1/1 -> Mux/1
  In1/1 -> Demux/1
  Subsystem Reference2/1 -> Mux/2
  Demux/2 -> Subsystem Reference2/1
  Demux/3 -> Subsystem Reference3/1
  Mux/1 -> Out1/1

== system DetailedModel/process measurements/DMA Averaging6 ==
  In1 : Inport
  Demux : Demux  Outputs=3
  Mux : Mux  Inputs=3
  Subsystem Reference1 : Subsystem  ReferencedSubsystem=DMA_frame_average  samplerate=h_BTU  framesize=DMA_framesize
  Subsystem Reference2 : Subsystem  ReferencedSubsystem=DMA_frame_average  samplerate=h_BTU  framesize=DMA_framesize
  Subsystem Reference3 : Subsystem  ReferencedSubsystem=DMA_frame_average  samplerate=h_BTU  framesize=DMA_framesize
  Out1 : Outport
  wires:
  Mux/1 -> Out1/1
  Demux/3 -> Subsystem Reference3/1
  Demux/2 -> Subsystem Reference2/1
  Subsystem Reference2/1 -> Mux/2
  In1/1 -> Demux/1
  Subsystem Reference1/1 -> Mux/1
  Subsystem Reference3/1 -> Mux/3
  Demux/1 -> Subsystem Reference1/1

== system DetailedModel/process measurements/DMA Averaging7 ==
  In1 : Inport
  Demux : Demux  Outputs=2
  Mux : Mux  Inputs=2
  Subsystem Reference1 : Subsystem  ReferencedSubsystem=DMA_frame_average  samplerate=h_BTU  framesize=DMA_framesize
  Subsystem Reference2 : Subsystem  ReferencedSubsystem=DMA_frame_average  samplerate=h_BTU  framesize=DMA_framesize
  u : Outport
  wires:
  Mux/1 -> u/1
  Demux/2 -> Subsystem Reference2/1
  Subsystem Reference2/1 -> Mux/2
  In1/1 -> Demux/1
  Subsystem Reference1/1 -> Mux/1
  Demux/1 -> Subsystem Reference1/1

== system DetailedModel/process measurements/DMA Averaging8 ==
  In1 : Inport
  Demux : Demux  Outputs=2
  Mux : Mux  Inputs=2
  Subsystem Reference1 : Subsystem  ReferencedSubsystem=DMA_frame_average  samplerate=h_BTU  framesize=DMA_framesize
  Subsystem Reference2 : Subsystem  ReferencedSubsystem=DMA_frame_average  samplerate=h_BTU  framesize=DMA_framesize
  u : Outport
  wires:
  Mux/1 -> u/1
  Demux/2 -> Subsystem Reference2/1
  Subsystem Reference2/1 -> Mux/2
  In1/1 -> Demux/1
  Subsystem Reference1/1 -> Mux/1
  Demux/1 -> Subsystem Reference1/1

== system DetailedModel/process measurements/DMA Averaging9 ==
  In1 : Inport
  Demux : Demux  Outputs=3
  Mux : Mux  Inputs=3
  Scope : Scope  Commented=on  NumInputPorts=3
  Scope1 : Scope  Commented=on  NumInputPorts=3
  Scope2 : Scope  Commented=on  NumInputPorts=3
  Subsystem Reference1 : Subsystem  ReferencedSubsystem=DMA_frame_average  samplerate=h_BTU  framesize=DMA_framesize
  Subsystem Reference2 : Subsystem  ReferencedSubsystem=DMA_frame_average  samplerate=h_BTU  framesize=DMA_framesize
  Subsystem Reference3 : Subsystem  ReferencedSubsystem=DMA_frame_average  samplerate=h_BTU  framesize=DMA_framesize
  Zero-Order Hold : ZeroOrderHold  Commented=on  SampleTime=h_BTU
  Zero-Order Hold1 : ZeroOrderHold  Commented=on  SampleTime=h_BTU
  Zero-Order Hold2 : ZeroOrderHold  Commented=on  SampleTime=h_BTU
  Zero-Order Hold3 : ZeroOrderHold  Commented=on  SampleTime=h_BTU/10
  Zero-Order Hold4 : ZeroOrderHold  Commented=on  SampleTime=h_BTU/10
  Zero-Order Hold5 : ZeroOrderHold  Commented=on  SampleTime=h_BTU/10
  u : Outport
  wires:
  Mux/1 -> u/1
  In1/1 -> Demux/1
  Subsystem Reference1/1 -> Scope/3, Mux/1
  Zero-Order Hold/1 -> Scope/2
  Demux/1 -> Zero-Order Hold3/1, Zero-Order Hold/1, Subsystem Reference1/1
  Subsystem Reference2/1 -> Scope1/3, Mux/2
  Demux/2 -> Zero-Order Hold4/1, Zero-Order Hold1/1, Subsystem Reference2/1
  Zero-Order Hold1/1 -> Scope1/2
  Subsystem Reference3/1 -> Scope2/3, Mux/3
  Demux/3 -> Zero-Order Hold2/1, Zero-Order Hold5/1, Subsystem Reference3/1
  Zero-Order Hold2/1 -> Scope2/2
  Zero-Order Hold3/1 -> Scope/1
  Zero-Order Hold4/1 -> Scope1/1
  Zero-Order Hold5/1 -> Scope2/1

== system DetailedModel/process measurements/HO_I_ABR_in ==
  u : Inport
  3ph HO Filter : Subsystem  VariantControl=Filter.I_ABR_in.HO.Mode
  Bypass : Subsystem  VariantControl=~Filter.I_ABR_in.HO.Mode
  y : Outport

== system DetailedModel/process measurements/HO_I_INV ==
  u : Inport
  3ph HO Filter : Subsystem  VariantControl=Filter.I_INV.HO.Mode
  Bypass : Subsystem  VariantControl=~Filter.I_INV.HO.Mode
  y : Outport

== system DetailedModel/process measurements/HO_I_LCL_Out ==
  u : Inport
  3ph HO Filter : Subsystem  VariantControl=Filter.I_LCL_Out.HO.Mode
  Bypass : Subsystem  VariantControl=~Filter.I_LCL_Out.HO.Mode
  y : Outport

== system DetailedModel/process measurements/HO_U_ABR_in ==
  u : Inport
  3ph HO Filter : Subsystem  VariantControl=Filter.U_ABR_in.HO.Mode
  Bypass : Subsystem  VariantControl=~Filter.U_ABR_in.HO.Mode
  y : Outport

== system DetailedModel/process measurements/HO_U_Grid_Out ==
  u : Inport
  3ph HO Filter : Subsystem  VariantControl=Filter.U_Grid_Out.HO.Mode
  Bypass : Subsystem  VariantControl=~Filter.U_Grid_Out.HO.Mode
  y : Outport

== system DetailedModel/process measurements/HO_U_INV ==
  u : Inport
  3ph HO Filter : Subsystem  VariantControl=Filter.U_INV.HO.Mode
  Bypass : Subsystem  VariantControl=~Filter.U_INV.HO.Mode
  y : Outport

== system DetailedModel/process measurements/HO_U_LCL_Out ==
  u : Inport
  3ph HO Filter : Subsystem  VariantControl=Filter.U_LCL_Out.HO.Mode
  Bypass : Subsystem  VariantControl=~Filter.U_LCL_Out.HO.Mode
  y : Outport

== system DetailedModel/process measurements/LO_I_DC ==
  u : Inport
  Bypass : Subsystem  VariantControl=~Filter.I_DC.LO.Mode
  Subsystem : Subsystem  VariantControl=Filter.I_DC.LO.Mode
  y : Outport

== system DetailedModel/process measurements/LO_U_DC ==
  u : Inport
  Bypass : Subsystem  VariantControl=~Filter.U_DC.LO.Mode
  Low_Order_Filter : Subsystem  VariantControl=Filter.U_DC.LO.Mode  ReferencedSubsystem=LO_Filter
  y : Outport

== system DetailedModel/process measurements/LO_U_DC_PosNeg ==
  u : Inport
  Bypass : Subsystem  VariantControl=~Filter.U_DC.LO.Mode
  Subsystem : Subsystem  VariantControl=Filter.U_DC.LO.Mode
  y : Outport

== system DetailedModel/IGBT Inverter/average model/For Each Subsystem ==
  In1 : Inport  Partition=on  PartitionDimension=1  PartitionWidth=1  PartitionOffset=0
  dc pos : Inport  Port=2
  dc neg : Inport  Port=3
  For Each : ForEach  DisableCoverage=on
  Product : Product
  Product1 : Product
  Switch : Switch  SaturateOnIntegerOverflow=off  InputSameDT=off
  Out1 : Outport  ConcatenationDimension=1
  wires:
  In1/1 -> Product1/1, Product/2, Switch/2
  Product/1 -> Switch/1
  dc pos/1 -> Product/1
  Product1/1 -> Switch/3
  dc neg/1 -> Product1/2
  Switch/1 -> Out1/1

== system DetailedModel/process measurements/HO_I_ABR_in/3ph HO Filter ==
  u : Inport
  Demux : Demux  Outputs=3
  High_Order_Filter_a : Subsystem  VariantControl=Filter.U_ABR_in.HO.Mode  ReferencedSubsystem=HO_Filter
  High_Order_Filter_b : Subsystem  VariantControl=Filter.U_ABR_in.HO.Mode  ReferencedSubsystem=HO_Filter
  High_Order_Filter_c : Subsystem  VariantControl=Filter.U_ABR_in.HO.Mode  ReferencedSubsystem=HO_Filter
  Mux : Mux  Inputs=3
  y : Outport
  wires:
  Demux/3 -> High_Order_Filter_c/1
  Demux/2 -> High_Order_Filter_b/1
  Demux/1 -> High_Order_Filter_a/1
  u/1 -> Demux/1
  Mux/1 -> y/1
  High_Order_Filter_a/1 -> Mux/1
  High_Order_Filter_c/1 -> Mux/3
  High_Order_Filter_b/1 -> Mux/2

== system DetailedModel/process measurements/HO_I_ABR_in/Bypass ==
  u : Inport
  y : Outport
  wires:
  u/1 -> y/1

== system DetailedModel/process measurements/HO_I_INV/3ph HO Filter ==
  u : Inport
  Demux : Demux  Outputs=3
  High_Order_Filter_a : Subsystem  VariantControl=Filter.U_ABR_in.HO.Mode  ReferencedSubsystem=HO_Filter
  High_Order_Filter_b : Subsystem  VariantControl=Filter.U_ABR_in.HO.Mode  ReferencedSubsystem=HO_Filter
  High_Order_Filter_c : Subsystem  VariantControl=Filter.U_ABR_in.HO.Mode  ReferencedSubsystem=HO_Filter
  Mux : Mux  Inputs=3
  y : Outport
  wires:
  Demux/3 -> High_Order_Filter_c/1
  Demux/2 -> High_Order_Filter_b/1
  Demux/1 -> High_Order_Filter_a/1
  u/1 -> Demux/1
  Mux/1 -> y/1
  High_Order_Filter_a/1 -> Mux/1
  High_Order_Filter_c/1 -> Mux/3
  High_Order_Filter_b/1 -> Mux/2

== system DetailedModel/process measurements/HO_I_INV/Bypass ==
  u : Inport
  y : Outport
  wires:
  u/1 -> y/1

== system DetailedModel/process measurements/HO_I_LCL_Out/3ph HO Filter ==
  u : Inport
  Demux : Demux  Outputs=3
  High_Order_Filter_a : Subsystem  VariantControl=Filter.U_ABR_in.HO.Mode  ReferencedSubsystem=HO_Filter
  High_Order_Filter_b : Subsystem  VariantControl=Filter.U_ABR_in.HO.Mode  ReferencedSubsystem=HO_Filter
  High_Order_Filter_c : Subsystem  VariantControl=Filter.U_ABR_in.HO.Mode  ReferencedSubsystem=HO_Filter
  Mux : Mux  Inputs=3
  y : Outport
  wires:
  High_Order_Filter_b/1 -> Mux/2
  High_Order_Filter_c/1 -> Mux/3
  High_Order_Filter_a/1 -> Mux/1
  Mux/1 -> y/1
  u/1 -> Demux/1
  Demux/1 -> High_Order_Filter_a/1
  Demux/2 -> High_Order_Filter_b/1
  Demux/3 -> High_Order_Filter_c/1

== system DetailedModel/process measurements/HO_I_LCL_Out/Bypass ==
  u : Inport
  y : Outport
  wires:
  u/1 -> y/1

== system DetailedModel/process measurements/HO_U_ABR_in/3ph HO Filter ==
  u : Inport
  Demux : Demux  Outputs=3
  High_Order_Filter_a : Subsystem  VariantControl=Filter.U_ABR_in.HO.Mode  ReferencedSubsystem=HO_Filter
  High_Order_Filter_b : Subsystem  VariantControl=Filter.U_ABR_in.HO.Mode  ReferencedSubsystem=HO_Filter
  High_Order_Filter_c : Subsystem  VariantControl=Filter.U_ABR_in.HO.Mode  ReferencedSubsystem=HO_Filter
  Mux : Mux  Inputs=3
  y : Outport
  wires:
  High_Order_Filter_b/1 -> Mux/2
  High_Order_Filter_c/1 -> Mux/3
  High_Order_Filter_a/1 -> Mux/1
  Mux/1 -> y/1
  u/1 -> Demux/1
  Demux/1 -> High_Order_Filter_a/1
  Demux/2 -> High_Order_Filter_b/1
  Demux/3 -> High_Order_Filter_c/1

== system DetailedModel/process measurements/HO_U_ABR_in/Bypass ==
  u : Inport
  y : Outport
  wires:
  u/1 -> y/1

== system DetailedModel/process measurements/HO_U_Grid_Out/3ph HO Filter ==
  u : Inport
  Demux : Demux  Outputs=3
  High_Order_Filter_a : Subsystem  VariantControl=Filter.U_ABR_in.HO.Mode  ReferencedSubsystem=HO_Filter
  High_Order_Filter_b : Subsystem  VariantControl=Filter.U_ABR_in.HO.Mode  ReferencedSubsystem=HO_Filter
  High_Order_Filter_c : Subsystem  VariantControl=Filter.U_ABR_in.HO.Mode  ReferencedSubsystem=HO_Filter
  Mux : Mux  Inputs=3
  y : Outport
  wires:
  High_Order_Filter_b/1 -> Mux/2
  High_Order_Filter_c/1 -> Mux/3
  High_Order_Filter_a/1 -> Mux/1
  Mux/1 -> y/1
  u/1 -> Demux/1
  Demux/1 -> High_Order_Filter_a/1
  Demux/2 -> High_Order_Filter_b/1
  Demux/3 -> High_Order_Filter_c/1

== system DetailedModel/process measurements/HO_U_Grid_Out/Bypass ==
  u : Inport
  y : Outport
  wires:
  u/1 -> y/1

== system DetailedModel/process measurements/HO_U_INV/3ph HO Filter ==
  u : Inport
  Demux : Demux  Outputs=3
  High_Order_Filter_a : Subsystem  VariantControl=Filter.U_ABR_in.HO.Mode  ReferencedSubsystem=HO_Filter
  High_Order_Filter_b : Subsystem  VariantControl=Filter.U_ABR_in.HO.Mode  ReferencedSubsystem=HO_Filter
  High_Order_Filter_c : Subsystem  VariantControl=Filter.U_ABR_in.HO.Mode  ReferencedSubsystem=HO_Filter
  Mux : Mux  Inputs=3
  y : Outport
  wires:
  Demux/3 -> High_Order_Filter_c/1
  Demux/2 -> High_Order_Filter_b/1
  Demux/1 -> High_Order_Filter_a/1
  u/1 -> Demux/1
  Mux/1 -> y/1
  High_Order_Filter_a/1 -> Mux/1
  High_Order_Filter_c/1 -> Mux/3
  High_Order_Filter_b/1 -> Mux/2

== system DetailedModel/process measurements/HO_U_INV/Bypass ==
  u : Inport
  y : Outport
  wires:
  u/1 -> y/1

== system DetailedModel/process measurements/HO_U_LCL_Out/3ph HO Filter ==
  u : Inport
  Demux : Demux  Outputs=3
  High_Order_Filter_a : Subsystem  VariantControl=Filter.U_ABR_in.HO.Mode  ReferencedSubsystem=HO_Filter
  High_Order_Filter_b : Subsystem  VariantControl=Filter.U_ABR_in.HO.Mode  ReferencedSubsystem=HO_Filter
  High_Order_Filter_c : Subsystem  VariantControl=Filter.U_ABR_in.HO.Mode  ReferencedSubsystem=HO_Filter
  Mux : Mux  Inputs=3
  y : Outport
  wires:
  High_Order_Filter_b/1 -> Mux/2
  High_Order_Filter_c/1 -> Mux/3
  High_Order_Filter_a/1 -> Mux/1
  Mux/1 -> y/1
  u/1 -> Demux/1
  Demux/1 -> High_Order_Filter_a/1
  Demux/2 -> High_Order_Filter_b/1
  Demux/3 -> High_Order_Filter_c/1

== system DetailedModel/process measurements/HO_U_LCL_Out/Bypass ==
  u : Inport
  y : Outport
  wires:
  u/1 -> y/1

== system DetailedModel/process measurements/LO_I_DC/Bypass ==
  u : Inport
  y : Outport
  wires:
  u/1 -> y/1

== system DetailedModel/process measurements/LO_I_DC/Subsystem ==
  u : Inport
  Demux : Demux  Outputs=2
  Low_Order_Filter : Subsystem  VariantControl=Filter.U_DC.LO.Mode  ReferencedSubsystem=LO_Filter
  Low_Order_Filter1 : Subsystem  VariantControl=Filter.U_DC.LO.Mode  ReferencedSubsystem=LO_Filter
  Mux : Mux  Inputs=2
  y : Outport
  wires:
  u/1 -> Demux/1
  Mux/1 -> y/1
  Low_Order_Filter/1 -> Mux/1
  Low_Order_Filter1/1 -> Mux/2
  Demux/1 -> Low_Order_Filter/1
  Demux/2 -> Low_Order_Filter1/1

== system DetailedModel/process measurements/LO_U_DC/Bypass ==
  u : Inport
  y : Outport
  wires:
  u/1 -> y/1

== system DetailedModel/process measurements/LO_U_DC_PosNeg/Bypass ==
  u : Inport
  y : Outport
  wires:
  u/1 -> y/1

== system DetailedModel/process measurements/LO_U_DC_PosNeg/Subsystem ==
  u : Inport
  Demux : Demux  Outputs=2
  Low_Order_Filter : Subsystem  VariantControl=Filter.U_DC.LO.Mode  ReferencedSubsystem=LO_Filter
  Low_Order_Filter1 : Subsystem  VariantControl=Filter.U_DC.LO.Mode  ReferencedSubsystem=LO_Filter
  Mux : Mux  Inputs=2
  y : Outport
  wires:
  u/1 -> Demux/1
  Mux/1 -> y/1
  Low_Order_Filter/1 -> Mux/1
  Low_Order_Filter1/1 -> Mux/2
  Demux/1 -> Low_Order_Filter/1
  Demux/2 -> Low_Order_Filter1/1

== matlab function DetailedModel/MATLAB Function ==
  data: t input; y output
function y = fcn(t)
t0 = 0.14;
width = 0.0015;
depth = 0.22;

if t < t0-width/2 || t > t0+width/2
    y = 1;
else
    y = 1 - depth*(cos((t-t0)*2*pi/width) + 1)/2;
end
